simulink model "Position_Controller_Design"  (R2024b)
settings: Solver=VariableStepAuto  StartTime=0.0  StopTime=10  RelTol=1e-3
values from neighbouring files (symbols this model uses):
  B = 0    [DC_Motor_Project.m]
  J = 0.00252    [DC_Motor_Project.m]
  K_as = 1/K_ps    (= 1.68552663541)    [DC_Motor_Project.m]
  K_ic = Ra * W_cc    (= 260)    [DC_Motor_Project.m]
  K_ip = 105.95*0.06418    (= 6.799871)    [DC_Motor_Project.m]
  K_is = (J* W_cs*W_cs) / (5 * Kt)    (= 11.8657276485)    [DC_Motor_Project.m]
  K_pc = La * W_cc    (= 1.7)    [DC_Motor_Project.m]
  K_pp = 105.95    [DC_Motor_Project.m]
  K_ps = J*W_cs / Kt    (= 0.593286382423)    [DC_Motor_Project.m]
  Kac = 1 / K_pc    (= 0.588235294118)    [DC_Motor_Project.m]
  Kt = Te_rated / Ia_rated    (= 0.424752712124)    [DC_Motor_Project.m]
  La = 1.7e-3    (= 0.0017)    [DC_Motor_Project.m]
  Ra = 0.26    [DC_Motor_Project.m]
settings Model: Creator=LEGION  LastModifiedBy=LEGION

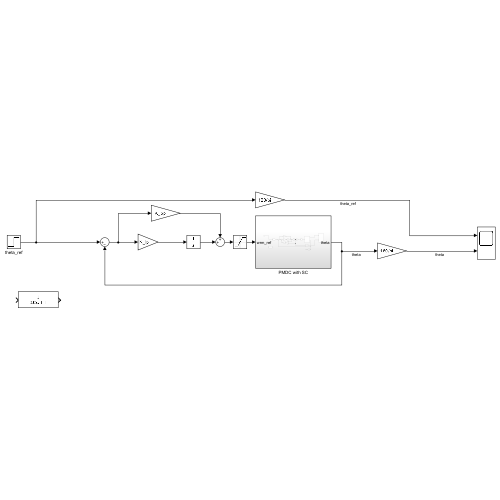
[thumbnail: Simulink's stored preview of the top-level diagram]
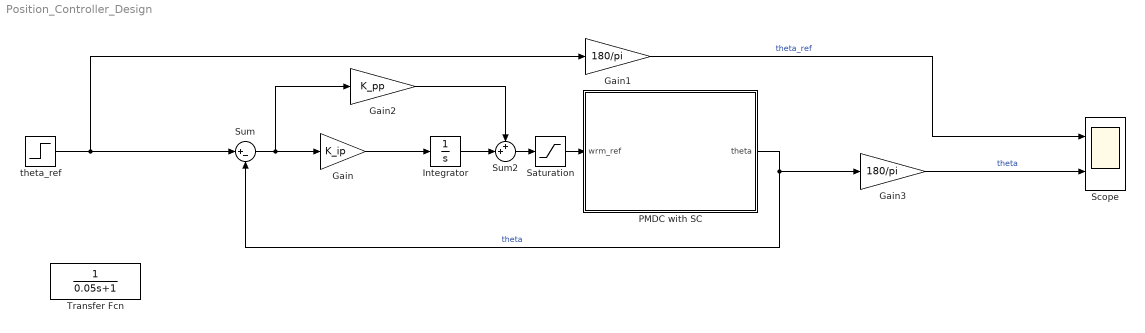
== system Position_Controller_Design ==
  Gain : Gain  Gain=K_ip
  Gain1 : Gain  Gain=180/pi
  Gain2 : Gain  Gain=K_pp
  Gain3 : Gain  Gain=180/pi
  Integrator : Integrator
  PMDC with SC : Subsystem
  Saturation : Saturate  UpperLimit=3000  LowerLimit=0
  Scope : Scope  NumInputPorts=2
  Sum : Sum  Inputs=|+-
  Sum2 : Sum  Inputs=++|
  Transfer Fcn : TransferFcn  Denominator=[0.05 1]
  theta_ref : Step  After=120 *pi/180  SampleTime=0
  wires:
  Gain/1 -> Integrator/1
  Sum/1 -> Gain2/1, Gain/1
  Integrator/1 -> Sum2/2
  Gain2/1 -> Sum2/1
  theta_ref/1 -> Sum/1, Gain1/1
  Sum2/1 -> Saturation/1
  PMDC with SC/1(theta) -> Sum/2, Gain3/1  "theta"
  Saturation/1 -> PMDC with SC/1(wrm_ref)
  Gain1/1 -> Scope/1  "theta_ref"
  Gain3/1 -> Scope/2  "theta"

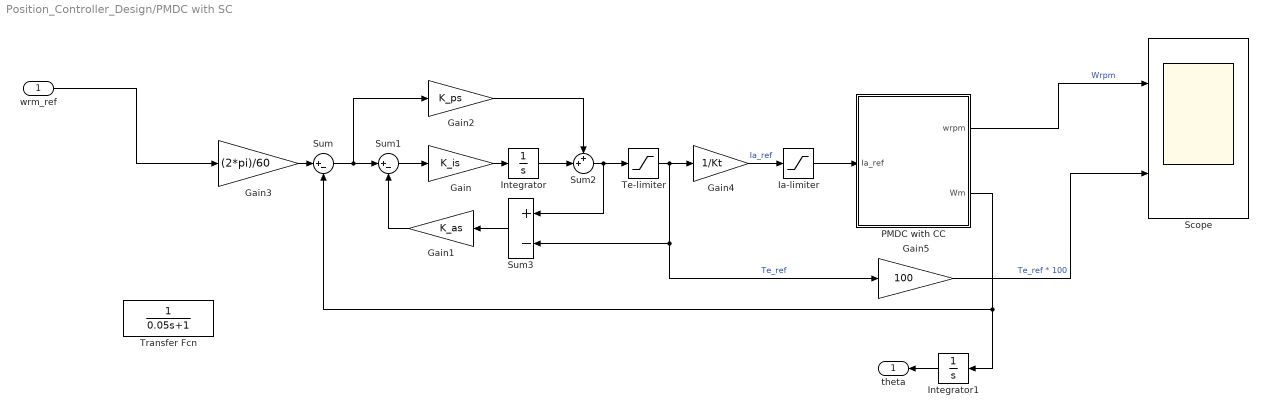
== system Position_Controller_Design/PMDC with SC ==
  wrm_ref : Inport
  Gain : Gain  Gain=K_is
  Gain1 : Gain  Gain=K_as
  Gain2 : Gain  Gain=K_ps
  Gain3 : Gain  Gain=(2*pi)/60
  Gain4 : Gain  Gain=1/Kt
  Gain5 : Gain  Gain=100
  Ia-limiter : Saturate  UpperLimit=25  LowerLimit=0
  Integrator : Integrator
  Integrator1 : Integrator
  PMDC with CC : Subsystem
  Scope : Scope  NumInputPorts=2
  Sum : Sum  Inputs=|+-
  Sum1 : Sum  Inputs=|+-
  Sum2 : Sum  Inputs=++|
  Sum3 : Sum  Inputs=+-
  Te-limiter : Saturate  UpperLimit=11  LowerLimit=-11
  Transfer Fcn : TransferFcn  Denominator=[0.05 1]
  theta : Outport
  wires:
  Gain4/1 -> Ia-limiter/1  "Ia_ref"
  Sum1/1 -> Gain/1
  Gain2/1 -> Sum2/1
  Sum3/1 -> Gain1/1
  Sum/1 -> Gain2/1, Sum1/1
  Te-limiter/1 -> Gain5/1, Sum3/2, Gain4/1  "Te_ref"
  PMDC with CC/2(Wm) -> Sum/2, Integrator1/1
  Gain5/1 -> Scope/2  "Te_ref * 100"
  Ia-limiter/1 -> PMDC with CC/1(Ia_ref)
  Integrator/1 -> Sum2/2
  Gain/1 -> Integrator/1
  Gain3/1 -> Sum/1
  PMDC with CC/1(wrpm) -> Scope/1  "Wrpm"
  Sum2/1 -> Sum3/1, Te-limiter/1
  Gain1/1 -> Sum1/2
  Integrator1/1 -> theta/1
  wrm_ref/1 -> Gain3/1

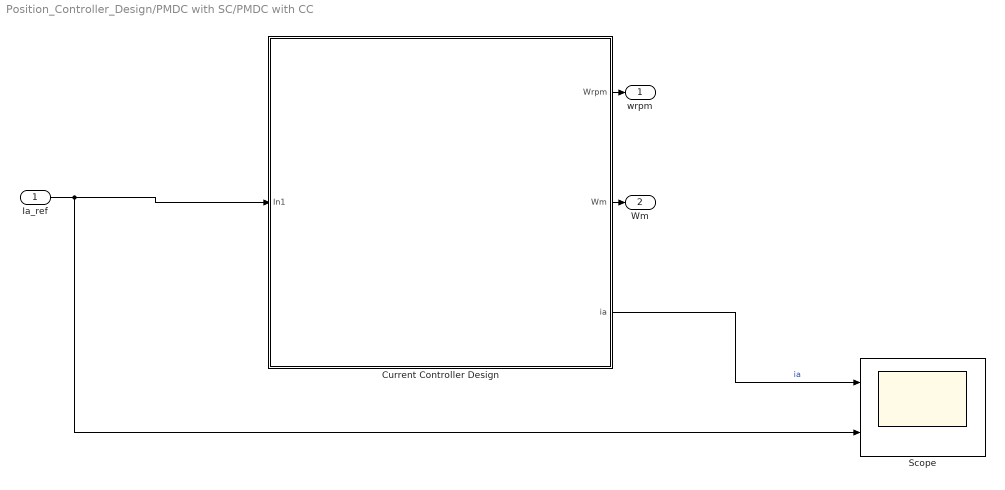
== system Position_Controller_Design/PMDC with SC/PMDC with CC ==
  Ia_ref : Inport
  Current Controller Design : Subsystem
  Scope : Scope  NumInputPorts=2
  wrpm : Outport
  Wm : Outport  Port=2
  wires:
  Current Controller Design/3(ia) -> Scope/1  "ia"
  Ia_ref/1 -> Scope/2, Current Controller Design/1(In1)
  Current Controller Design/1(Wrpm) -> wrpm/1
  Current Controller Design/2(Wm) -> Wm/1

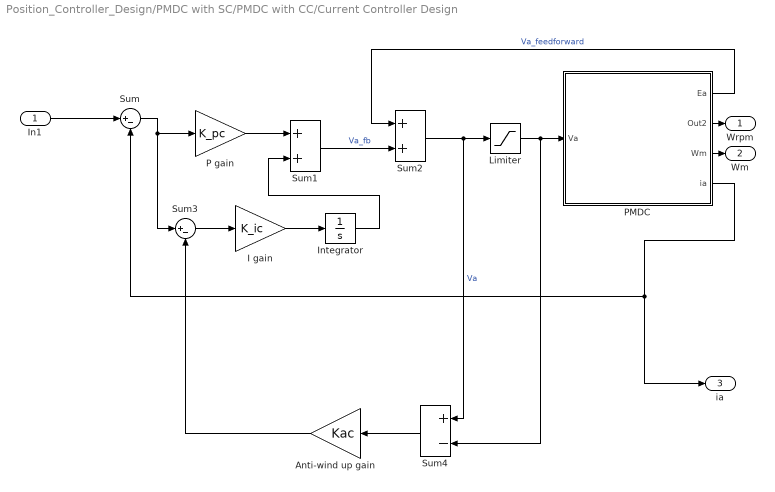
== system Position_Controller_Design/PMDC with SC/PMDC with CC/Current Controller Design ==
  In1 : Inport
  Anti-wind up gain : Gain  Gain=Kac
  I gain : Gain  Gain=K_ic
  Integrator : Integrator
  Limiter : Saturate  UpperLimit=140  LowerLimit=0
  P gain : Gain  Gain=K_pc
  PMDC : Subsystem
  Sum : Sum  Inputs=|+-
  Sum1 : Sum
  Sum2 : Sum
  Sum3 : Sum  Inputs=|+-
  Sum4 : Sum  Inputs=+-
  Wrpm : Outport
  Wm : Outport  Port=2
  ia : Outport  Port=3
  wires:
  PMDC/4(ia) -> ia/1, Sum/2
  Integrator/1 -> Sum1/2
  Sum/1 -> Sum3/1, P gain/1
  I gain/1 -> Integrator/1
  Anti-wind up gain/1 -> Sum3/2
  P gain/1 -> Sum1/1
  Limiter/1 -> Sum4/2, PMDC/1(Va)
  In1/1 -> Sum/1
  Sum4/1 -> Anti-wind up gain/1
  PMDC/1(Ea) -> Sum2/1  "Va_feedforward"
  Sum1/1 -> Sum2/2  "Va_fb"
  Sum3/1 -> I gain/1
  Sum2/1 -> Sum4/1, Limiter/1  "Va"
  PMDC/2(Out2) -> Wrpm/1
  PMDC/3(Wm) -> Wm/1

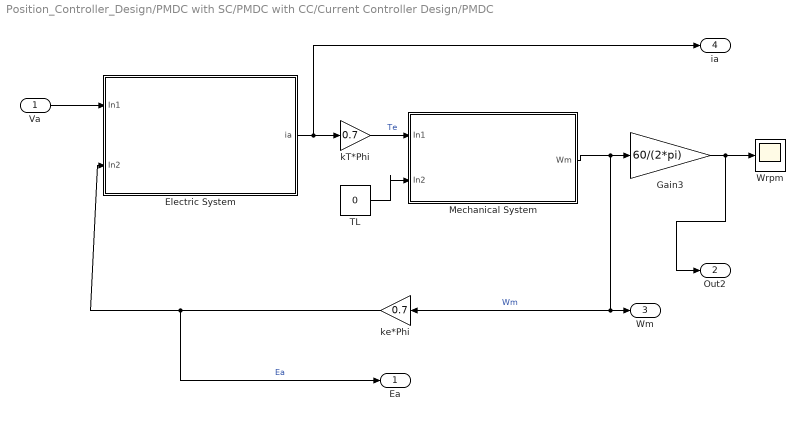
== system Position_Controller_Design/PMDC with SC/PMDC with CC/Current Controller Design/PMDC ==
  Va : Inport
  Electric System : Subsystem
  Gain3 : Gain  Gain=60/(2*pi)
  Mechanical System : Subsystem
  TL : Constant  Value=0
  Wrpm : Scope
  kT*Phi : Gain  Gain=0.7
  ke*Phi : Gain  Gain=0.7
  Ea : Outport
  Out2 : Outport  Port=2
  Wm : Outport  Port=3
  ia : Outport  Port=4
  wires:
  ke*Phi/1 -> Ea/1, Electric System/2(In2)  "Ea"
  kT*Phi/1 -> Mechanical System/1(In1)  "Te"
  Mechanical System/1(Wm) -> Wm/1, ke*Phi/1, Gain3/1  "Wm"
  Gain3/1 -> Out2/1, Wrpm/1
  Electric System/1(ia) -> ia/1, kT*Phi/1
  TL/1 -> Mechanical System/2(In2)
  Va/1 -> Electric System/1(In1)

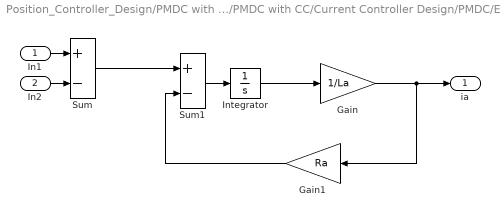
== system Position_Controller_Design/PMDC with SC/PMDC with CC/Current Controller Design/PMDC/Electric System ==
  In1 : Inport
  In2 : Inport  Port=2
  Gain : Gain  Gain=1/La
  Gain1 : Gain  Gain=Ra
  Integrator : Integrator
  Sum : Sum  Inputs=+-
  Sum1 : Sum  Inputs=+-
  ia : Outport
  wires:
  Sum1/1 -> Integrator/1
  In1/1 -> Sum/1
  Gain1/1 -> Sum1/2
  Gain/1 -> ia/1, Gain1/1
  Sum/1 -> Sum1/1
  Integrator/1 -> Gain/1
  In2/1 -> Sum/2

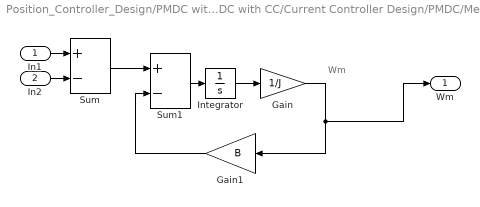
== system Position_Controller_Design/PMDC with SC/PMDC with CC/Current Controller Design/PMDC/Mechanical System ==
  note: Wm
  In1 : Inport
  In2 : Inport  Port=2
  Gain : Gain  Gain=1/J
  Gain1 : Gain  Gain=B
  Integrator : Integrator
  Sum : Sum  Inputs=+-
  Sum1 : Sum  Inputs=+-
  Wm : Outport
  wires:
  Gain/1 -> Wm/1, Gain1/1
  Sum1/1 -> Integrator/1
  Sum/1 -> Sum1/1
  In1/1 -> Sum/1
  Gain1/1 -> Sum1/2
  Integrator/1 -> Gain/1
  In2/1 -> Sum/2
